simulink model "windPlantAvg"  (R2026a)
settings: Solver=ode23tb  StopTime=30  MaxStep=0.01  RelTol=1e-4  AbsTol=1e-6
model workspace (MATLAB code in the model file):
  | wp = windParams();
  | wp = rmfield(wp, {'li_inv','Cp'});   % handles: not usable inside a block
libraries: windLib x2
Description:
  | Wind branch, AVERAGED fidelity (controller tuning, scenario harness, SCR sweep).
  | 30 kW PMSG -> 3-phase diode bridge -> boost + MPPT, feeding its own DC link (DC link 2)
  | and grid-tie inverter. AC-coupled architecture per the product-owner meeting of 3 Sep 2026 (30 kW is the team's rating).
  | Every parameter comes from params/windParams.m via the model workspace - no constants in masks.
  | Aerodynamics and MPPT are library links to windLib.slx. Owner: Ba Huy Ta.
settings Model: Creator=huyta  LastModifiedBy=huyta

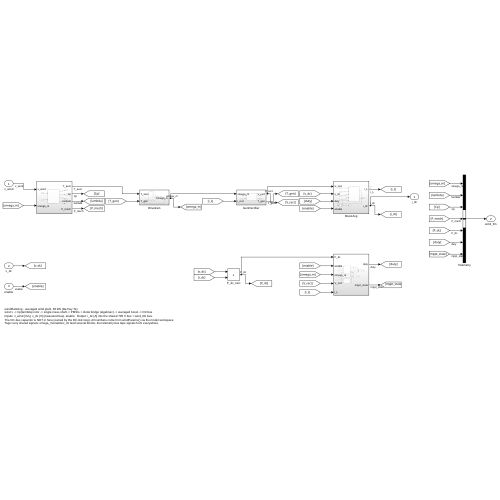
[thumbnail: Simulink's stored preview of the top-level diagram]
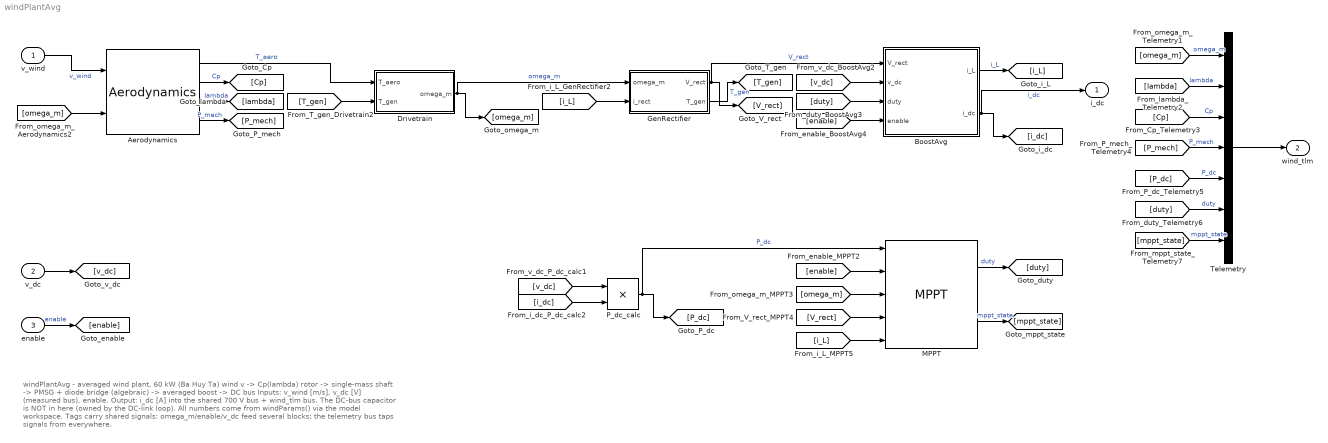
== system windPlantAvg ==
  note: windPlantAvg - averaged wind plant, 60 kW (Ba Huy Ta)
      | wind v -> Cp(lambda) rotor -> single-mass shaft -> PMSG + diode bridge (algebraic) -> averaged boost -> DC bus
      | Inputs: v_wind [m/s], v_dc [V] (measured bus), enable.  Output: i_dc [A] into the shared 700 V bus + wind_tlm bus.
      | The DC-bus capacitor is NOT in here (owned by the DC-link loop). All numbers come from windParams() via the model workspace.
      | Tags carry shared signals: omega_m/enable/v_dc feed several blocks; the telemetry bus taps signals from everywhere.
  v_wind : Inport
  v_dc : Inport  Port=2
  enable : Inport  Port=3
  Aerodynamics : windLib/Aerodynamics  SystemSampleTime=-1  VariantActivationTime=update diagram  EmptyChoice=off  PassThrough=off  PassThroughVariantControl=(default)  EmptyChoiceVariantControl=(default)  AllowFlexibleInterface=on  Latency=0  AutoFrameSizeCalculation=off
  BoostAvg : Subsystem
  Drivetrain : Subsystem
  GenRectifier : Subsystem
  MPPT : windLib/MPPT  SystemSampleTime=-1  VariantActivationTime=update diagram  EmptyChoice=off  PassThrough=off  PassThroughVariantControl=(default)  EmptyChoiceVariantControl=(default)  AllowFlexibleInterface=on  Latency=0  AutoFrameSizeCalculation=off
  P_dc_calc : Product
  Telemetry : BusCreator  Inputs=7
  i_dc : Outport
  wind_tlm : Outport  Port=2
  wires:
  MPPT/2 -> [mppt_state]  "mppt_state"
  [mppt_state] -> Telemetry/7  "mppt_state"
  MPPT/1 -> [duty]  "duty"
  [duty] -> Telemetry/6  "duty"
  [duty] -> BoostAvg/3(duty)
  Aerodynamics/4 -> [P_mech]  "P_mech"
  [P_mech] -> Telemetry/4  "P_mech"
  Aerodynamics/2 -> [Cp]  "Cp"
  [Cp] -> Telemetry/3  "Cp"
  Aerodynamics/3 -> [lambda]  "lambda"
  [lambda] -> Telemetry/2  "lambda"
  Aerodynamics/1 -> Drivetrain/1(T_aero)  "T_aero"
  v_wind/1 -> Aerodynamics/1  "v_wind"
  BoostAvg/2(i_dc) -> [i_dc], i_dc/1  "i_dc"
  [i_dc] -> P_dc_calc/2
  enable/1 -> [enable]  "enable"
  [enable] -> MPPT/2
  [enable] -> BoostAvg/4(enable)
  GenRectifier/1(V_rect) -> [V_rect], BoostAvg/1(V_rect)  "V_rect"
  [V_rect] -> MPPT/4
  BoostAvg/1(i_L) -> [i_L]  "i_L"
  [i_L] -> MPPT/5
  [i_L] -> GenRectifier/2(i_rect)
  GenRectifier/2(T_gen) -> [T_gen]  "T_gen"
  [T_gen] -> Drivetrain/2(T_gen)
  Drivetrain/1(omega_m) -> [omega_m], GenRectifier/1(omega_m)  "omega_m"
  [omega_m] -> MPPT/3
  [omega_m] -> Aerodynamics/2
  [omega_m] -> Telemetry/1  "omega_m"
  Telemetry/1 -> wind_tlm/1
  P_dc_calc/1 -> [P_dc], MPPT/1  "P_dc"
  [P_dc] -> Telemetry/5  "P_dc"
  v_dc/1 -> [v_dc]
  [v_dc] -> P_dc_calc/1
  [v_dc] -> BoostAvg/2(v_dc)

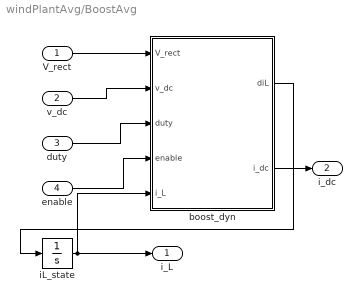
== system windPlantAvg/BoostAvg ==
  V_rect : Inport
  v_dc : Inport  Port=2
  duty : Inport  Port=3
  enable : Inport  Port=4
  boost_dyn : MATLAB Function  TreatAsAtomicUnit=on
  iL_state : Integrator  InitialCondition=wp.iL_init  LimitOutput=on  LowerSaturationLimit=0
  i_L : Outport
  i_dc : Outport  Port=2
  wires:
  boost_dyn/1(diL) -> iL_state/1
  enable/1 -> boost_dyn/4(enable)
  iL_state/1 -> i_L/1, boost_dyn/5(i_L)
  duty/1 -> boost_dyn/3(duty)
  v_dc/1 -> boost_dyn/2(v_dc)
  boost_dyn/2(i_dc) -> i_dc/1
  V_rect/1 -> boost_dyn/1(V_rect)

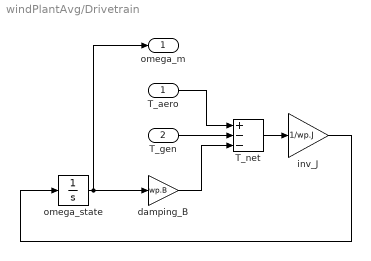
== system windPlantAvg/Drivetrain ==
  T_aero : Inport
  T_gen : Inport  Port=2
  T_net : Sum  Inputs=+--
  damping_B : Gain  Gain=wp.B
  inv_J : Gain  Gain=1/wp.J
  omega_state : Integrator  InitialCondition=wp.w_init  LimitOutput=on  LowerSaturationLimit=0.1
  omega_m : Outport
  wires:
  T_net/1 -> inv_J/1
  damping_B/1 -> T_net/3
  T_gen/1 -> T_net/2
  T_aero/1 -> T_net/1
  inv_J/1 -> omega_state/1
  omega_state/1 -> damping_B/1, omega_m/1

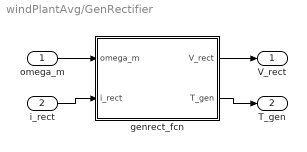
== system windPlantAvg/GenRectifier ==
  omega_m : Inport
  i_rect : Inport  Port=2
  genrect_fcn : MATLAB Function  TreatAsAtomicUnit=on
  V_rect : Outport
  T_gen : Outport  Port=2
  wires:
  genrect_fcn/2(T_gen) -> T_gen/1
  genrect_fcn/1(V_rect) -> V_rect/1
  i_rect/1 -> genrect_fcn/2(i_rect)
  omega_m/1 -> genrect_fcn/1(omega_m)

== matlab function windPlantAvg/GenRectifier/genrect_fcn ==
  data: omega_m input; V_rect output; i_rect input; T_gen output; wp parameter
function [V_rect, T_gen] = genrect_fcn(omega_m, i_rect, wp)
%#codegen
% PMSG + 3-phase uncontrolled diode bridge, collapsed to its averaged DC form.
%
% The open-circuit relation V_dc = 1.35*V_ll is only the starting point. The
% loading terms below are what stop the bridge behaving like an ideal source -
% without them the MPPT has nothing to hunt against and the result flatters.

w = max(omega_m, 0.1);
i = max(i_rect,  0);        % a diode bridge conducts one way only

w_e  = wp.p*w;                    % electrical rad/s
E_pk = w_e*wp.lam_pm;             % per-phase peak back-EMF
V_ll = E_pk*sqrt(3)/sqrt(2);      % line-to-line rms
V_oc = 1.35*V_ll;                 % ideal 6-pulse rectified voltage

V_rect = V_oc ...
         - (3/pi)*w_e*wp.Ls*i ...    % commutation overlap (source inductance)
         - 2*wp.Rs*i ...             % two phases conducting in series
         - wp.V_f;                   % two diode forward drops
V_rect = max(V_rect, 0);

% Shaft torque must account for ALL power leaving the machine, including the
% losses above - otherwise the drivetrain gets energy for free.
P_gen = V_rect*i + 2*wp.Rs*i^2 + wp.V_f*i;
T_gen = P_gen/w;
end

== matlab function windPlantAvg/BoostAvg/boost_dyn ==
  data: V_rect input; diL output; v_dc input; duty input; enable input; i_L input; i_dc output; wp parameter
function [diL, i_dc] = boost_dyn(V_rect, v_dc, duty, enable, i_L, wp)
%#codegen
% State-space averaged (switching-function) boost converter.
% One state, the inductor current; the switching ripple is deliberately not
% represented - that is what the switched variant is for.

% Duty limits belong to the plant, not the controller: the converter cannot
% exceed them no matter what the MPPT asks for.
d = min(max(duty, wp.d_min), wp.duty_max);
if enable <= 0.5
    d = 0;
end

i = max(i_L, 0);
diL = (V_rect - (1 - d)*v_dc - wp.R_L*i)/wp.L_boost;

% Unidirectional: the boost diode cannot pull current back out of the bus, so
% the current sticks at zero rather than reversing (discontinuous conduction).
if i <= 0 && diL < 0
    diL = 0;
end

% Current delivered to the shared 700 V DC bus.
i_dc = (1 - d)*i;
if enable <= 0.5
    i_dc = 0;
end
end
